simulink model "MotorDriveThermalTestbench"  (R2024b)
settings: Solver=daessc  StartTime=0.0  StopTime=2400  FixedStep=dt  RelTol=1e-3  AbsTol=1e-3
PreLoadFcn:
  | % Simulation parameters
  | MotorDriveThermalTestBenchParams;
model workspace (MAT data in the model file):
  V_frac_bridge = 0.0437
  V_fract_teeth = 0.9563
values from neighbouring files (symbols this model uses):
  CaseParams = struct()    [InverterThermalParams.m]
  HeatsinkParams = struct()    [InverterThermalParams.m]
undefined symbols (not defined in the file or in its folder): electricDrive, H_AH, H_AL, H_BH, H_BL, H_CH, H_CL, PipeParams, vehicleThermal
libraries: fl_lib x171, ee_lib x31, nesl_utility x28, nesl_utility_internal x12, sdl_lib x6, SimscapeFluids_lib x3, autolibshared x1
(part 1 of 4)
Description:
  | Copyright 2022 - 2023 The MathWorks, Inc.
settings Model: Creator=The MathWorks, Inc.  LastModifiedBy=jjha
settings SolverCC: AutoScaleAbsTol=off  InitialStep=1e-3  MaxConsecutiveMinStep=100  AlgebraicLoopSolver=TrustRegion
settings DataIOCC: MaxDataPoints=30000  SaveFormat=Array  SignalLoggingName=logsoutPMSMThermalTestbench  ReturnWorkspaceOutputsName=simoutPmsmThermalTestbench
settings OptimizationCC: BlockReduction=off  BooleanDataType=off  ReuseModelBlockBuffer=off  LifeSpan=inf
settings DebuggingCC: SaveWithParameterizedLinksMsg=none  SignalResolutionControl=TryResolveAllWithWarning  UnconnectedInputMsg=warning  UnconnectedOutputMsg=warning  UnconnectedLineMsg=warning  AllowSymbolicDim=off  SFUnexpectedBacktrackingDiag=warning  SFNoUnconditionalDefaultTransitionDiag=warning  SFExecutionAtInitializationDiag=none  ArithmeticOperatorsInVariantConditions=warning
settings HardwareCC: ProdBitPerPointer=32  ProdBitPerSizeT=32  ProdBitPerPtrDiffT=32  ProdLargestAtomicFloat=None  ProdIntDivRoundTo=Undefined  ProdEndianess=Unspecified  ProdWordSize=32  ProdHWDeviceType=32-bit Generic  TargetUnknown=on
settings ModelReferenceCC: EnableRefExpFcnMdlSchedulingChecks=on  PropagateSignalLabelsOutOfModel=off
settings SFSimCC: SimUseLocalCustomCode=off  CustomCodeUndefinedFunction=UseInterfaceOnly
settings RTWCC: RTWUseLocalCustomCode=off  GPUComputeCapability=3.5  DLArmComputeVersion=19.05
settings CodeAppCC: StateflowObjectComments=on
settings GRTTargetCC: TargetLangStandard=C89/C90 (ANSI)
settings ConfigComp: CovMetricSettings=dw  CovSaveCumulativeToWorkspaceVar=on  CovSaveSingleToWorkspaceVar=on  CovExternalEMLEnable=off  CovSFcnEnable=off
settings SimscapeCC: SimscapeLogType=all  SimscapeLogSimulationStatistics=on  SimscapeLogName=simlogPmsmThermalTestbench  SimscapeLogLimitData=off  SimscapeLogDataHistory=30000

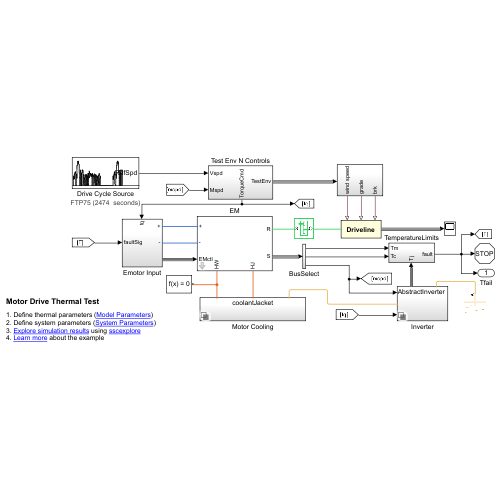
[thumbnail: Simulink's stored preview of the top-level diagram]
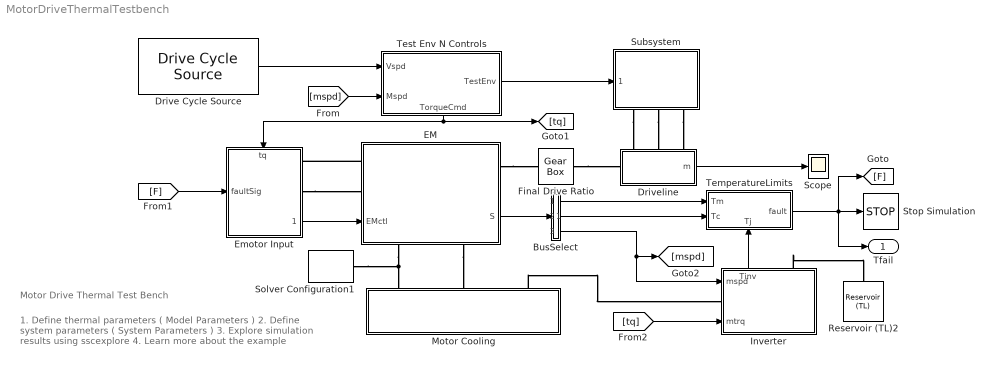
== system MotorDriveThermalTestbench ==
  note: Motor Drive Thermal Test Bench
  note: 1. Define thermal parameters ( Model Parameters )
      | 2. Define system parameters ( System Parameters )
      | 3. Explore simulation results using sscexplore
      | 4. Learn more about the example
  BusSelect : Subsystem
  Drive Cycle Source : autolibshared/Drive Cycle Source  cycleVar=FTP75  wsVar=LSHT  fileVar=cycleFTP75.mat  tfinal="2474  seconds"  cycleRepeat=off  outAccPort=off  outGearPort=off  gearList=No gear data  t_wot1=5  xdot_woto=0  xdot_wot1=30  t_wot2=20  xdot_wot2=0  t_wotend=30  srcUnit=m/s  outUnit=km/h  srcAccUnit=m/s/s  outAccUnit=m/s^2  dt=0  aMode=1  faultOption=off  velBnd=2  velBndUnit=mph  inUnit=m/s  timeBnd=1  failOption=off  stopSim=off  maxFaultCnt=10  maxFaultTime=2  maxTotFaultTime=15  traceOption=off  dtTrace=1  traceWindow=10  lastDCname=FTP75  lastOutUnit=mph  lastDT=0  lastTB=1  lastSB=2  forceCalcBound=off
  Driveline : Subsystem
      settings: PortSchema="{\"entries\":[{\"content\":{\"sides\":[{\"content\":{\"connectorIds\":[\"Out1\"]},\"type\":\"ConnectorPlacement.EquallySpacedRectSide\",\"uuid\":\"f321ff85-78a4-45a4-ab97-f20c5abfaf5e\"},{\"content\":{\"connectorIds\":[\"RConn1\"],\"side\":\"RIGHT\"},\"type\":\"ConnectorPlacement.EquallySpacedRectSide\",\"uuid\":\"2baf3540-3ef2-4140-8c68-0a1895e3ee25\"},{\"content\":{\"connectorIds\":[\"LConn1\",\"LConn2\",\"LConn3\"],\"side\":\"TOP\"},\"type\":\"ConnectorPlacement.EquallySpacedRectSide\",\"uuid\":\"1e5b09ba-71c5-41d6-b265-2fb2d783e941\"}]},\"type\":\"ConnectorPlacement.EquallySpacedConnector\",\"uuid\":\"4c01441a-ee4a-4858-900a-4caacc6910c3\"}],\"packageUris\":[\"http://schema.mathworks.com/mf0/Connector/R2020b\"],\"version\":\"1.0\"}"
      mask Display:
      | %disp(get_param(gcb, 'Name'))
      | disp(['{\bf\fontsize{12}' get_param(gcb, 'Name') '}'], 'texmode','on');
  EM : Subsystem  mask{InitTemp=vehicleThermal.coolant_T_init, IronSpHeat=electricDrive.IronSpHeat, CopperSpHeat=electricDrive.CopperSpHeat, IronThConductivity=electricDrive.IronThConductivity, GrossToothMass=electricDrive.MotorThermal.GrossToothMass, WindingMass=electricDrive.MotorThermal.WindingMass, max_torque=electricDrive.max_torque, max_power=electricDrive.max_power, Tctc=electricDrive.Tctc, spMat=electricDrive.motor_loss_map.spMat, tqMat=electricDrive.motor_loss_map.tqMat, lossMat=electricDrive.motor_loss_map.lossMat, StatorBackIronMass=electricDrive.MotorThermal.StatorBackIronMass, StatorRootDia=electricDrive.MotorThermal.StatorRootDia, stator_od=electricDrive.MotorThermal.stator_od, StatorWindingOhArea=electricDrive.MotorThermal.StatorWindingOhArea, Bridgemass=electricDrive.MotorThermal.Bridgemass, rotor_od=electricDrive.MotorThermal.rotor_od, rotorStackLength=electricDrive.MotorThermal.rotorStackLength, RotorBackIronMass=electricDrive.MotorThermal.RotorBackIronMass, RotorAreaER=electricDrive.MotorThermal.RotorAreaER, RotorAreaCyl=electricDrive.MotorThermal.RotorAreaCyl}
      mask prompts: InitTemp "Initial Temperature(K)"; IronSpHeat "Specific Heat Iron(J/(K*kg))"; CopperSpHeat "Specific Heat Copper(J/(K*kg))"; IronThConductivity "Thermal Conductivity Iron(W/(K*m))"; GrossToothMass "Stator Teeth Mass(kg)"; WindingMass "Stator Winding Mass(kg)"; max_torque "Max Torque"; max_power "Max Power"; Tctc "Torque Control Time Constant"; spMat "Speed Vector (rpm)"; tqMat "TorqueVector (Nm)"; lossMat "Losses (W)"; StatorBackIronMass "Stator Back Iron Mass(kg)"; StatorRootDia "Stator Inner Diameter (m)"; stator_od "Stator Outer Diameter(m)"; StatorWindingOhArea "Stator Winding Area(m^2)"; Bridgemass "Magnet Mass(kg)"; rotor_od "Rotor Outer Diameter(m)"; rotorStackLength "Stack Length(m)"; RotorBackIronMass "Rotor Iron Mass(kg)"; RotorAreaER "Rotor Area ER(m^2)"; RotorAreaCyl "Rotor Cylinder Area(m^2)"
      settings: LibrarySourceBlock=EmotorLib/Emotor Thermal  PortSchema="{\"entries\":[{\"content\":{\"sides\":[{\"content\":{\"connectorIds\":[\"LConn1\",\"LConn2\",\"In1\"]},\"type\":\"ConnectorPlacement.EquallySpacedRectSide\",\"uuid\":\"10df522d-563d-4b08-8533-b994fdc6485c\"},{\"content\":{\"connectorIds\":[\"RConn1\",\"Out1\"],\"side\":\"RIGHT\"},\"type\":\"ConnectorPlacement.EquallySpacedRectSide\",\"uuid\":\"49c7f672-865f-471b-9e0c-89a8670e12b9\"},{\"content\":{\"connectorIds\":[],\"side\":\"TOP\"},\"type\":\"ConnectorPlacement.EquallySpacedRectSide\",\"uuid\":\"483d1bb0-f2a2-4e3e-b03d-59043e33c561\"},{\"content\":{\"connectorIds\":[\"RConn2\",\"RConn3\"],\"side\":\"BOTTOM\"},\"type\":\"ConnectorPlacement.EquallySpacedRectSide\",\"uuid\":\"9824884f-8ef8-4acd-9b94-f9f251c18df1\"}]},\"type\":\"ConnectorPlacement.EquallySpacedConnector\",\"uuid\":\"fbb57d51-9a3c-403f-b1bb-2fd61ef310af\"}],\"packageUris\":[\"http://schema.mathworks.com/mf0/Connector/R2020b\"],\"version\":\"1.0\"}"
      mask DialogControl Container5 Prompt: Electrical Parameters
      mask DialogControl ElecTorque Prompt: Electrical Torque Parameters
      mask DialogControl ElecLosses Prompt: Electrical Losses Parameter
      mask DialogControl Container6 Prompt: Thermal Parameters
      mask DialogControl Container8 Prompt: Rotor
      mask DialogControl Container7 Prompt: Stator
  Emotor Input : Subsystem
      settings: PortSchema="{\"entries\":[{\"content\":{\"sides\":[{\"content\":{\"connectorIds\":[\"In1\"]},\"type\":\"ConnectorPlacement.EquallySpacedRectSide\",\"uuid\":\"c4c07ff1-e6b7-44ff-b3a5-b0e10b4cc465\"},{\"content\":{\"connectorIds\":[\"RConn1\",\"RConn2\",\"Out1\"],\"side\":\"RIGHT\"},\"type\":\"ConnectorPlacement.EquallySpacedRectSide\",\"uuid\":\"925c4aa1-6eb7-46da-8525-6fdd9359c532\"},{\"content\":{\"connectorIds\":[\"In2\"],\"side\":\"TOP\"},\"type\":\"ConnectorPlacement.EquallySpacedRectSide\",\"uuid\":\"640b893a-14a3-4b76-a9bc-18e7c0276558\"}]},\"type\":\"ConnectorPlacement.EquallySpacedConnector\",\"uuid\":\"1af614e2-1b17-4f3a-ad07-bd248b373d7b\"}],\"packageUris\":[\"http://schema.mathworks.com/mf0/Connector/R2020b\"],\"version\":\"1.0\"}"
  Final Drive Ratio : fl_lib/Mechanical/Mechanisms/Gear Box  ratio=electricDrive.VehicleParams.Gear_ratio  t_in_specify=off  t_in_priority=High  t_in=0 N*m  t_in_nominal_specify=off  t_in_nominal_value=1  t_in_nominal_unit=N*m  t_out_specify=off  t_out_priority=High  t_out=0 N*m  t_out_nominal_specify=off  t_out_nominal_value=1  t_out_nominal_unit=N*m
  Inverter : Subsystem  Variant=on  VariantControlMode=label  LabelModeActiveChoice=AbstractOn
      settings: PortSchema="{\"entries\":[{\"content\":{\"sides\":[{\"content\":{\"connectorIds\":[\"In1\",\"LConn1\",\"In2\"]},\"type\":\"ConnectorPlacement.EquallySpacedRectSide\",\"uuid\":\"633c2257-0ab1-4a3f-bc19-db971bbd7d23\"},{\"content\":{\"connectorIds\":[],\"side\":\"RIGHT\"},\"type\":\"ConnectorPlacement.EquallySpacedRectSide\",\"uuid\":\"268aca27-453a-4262-b99b-2b00bb036744\"},{\"content\":{\"connectorIds\":[\"Out1\",\"LConn2\"],\"side\":\"TOP\"},\"type\":\"ConnectorPlacement.EquallySpacedRectSide\",\"uuid\":\"94eb7410-69a0-4bb3-bfbc-11fdf2441086\"}]},\"type\":\"ConnectorPlacement.EquallySpacedConnector\",\"uuid\":\"4856a95d-ab29-4fb1-a283-1ba036af507a\"}],\"packageUris\":[\"http://schema.mathworks.com/mf0/Connector/R2020b\"],\"version\":\"1.0\"}"
  Motor Cooling : Subsystem  Variant=on  VariantControlMode=label  LabelModeActiveChoice=JacketOn
      settings: PortSchema="{\"entries\":[{\"content\":{\"sides\":[{\"content\":{\"connectorIds\":[]},\"type\":\"ConnectorPlacement.EquallySpacedRectSide\",\"uuid\":\"fad2e2e2-c8a8-4ae7-a5e0-e2d04801ad81\"},{\"content\":{\"connectorIds\":[],\"side\":\"RIGHT\"},\"type\":\"ConnectorPlacement.EquallySpacedRectSide\",\"uuid\":\"a876eae4-26d9-44a3-9dd3-410a35dafbf1\"},{\"content\":{\"connectorIds\":[\"LConn1\",\"LConn2\",\"LConn3\"],\"side\":\"TOP\"},\"type\":\"ConnectorPlacement.EquallySpacedRectSide\",\"uuid\":\"b2d352a8-e78b-4f23-87e4-b1c134d4f518\"}]},\"type\":\"ConnectorPlacement.EquallySpacedConnector\",\"uuid\":\"4da0a1ca-7739-4d5f-a9bc-f50bcf2d911d\"}],\"packageUris\":[\"http://schema.mathworks.com/mf0/Connector/R2020b\"],\"version\":\"1.0\"}"
  Reservoir (TL)2 : fl_lib/Thermal Liquid/Elements/Reservoir (TL)  pressure_spec=foundation.enum.pressure_spec.atmospheric  reservoir_pressure=0.101325 MPa  reservoir_temperature=TankParams.Temp K  area=0.01 m^2
  Scope : Scope
  Solver Configuration1 : nesl_utility/Solver Configuration  PhysicalDomain=network_engine_domain  SubClassName=solver  LeftPortType=input  RightPortType=generic  Tones=[]  Harmonics=[]  SimulateNoise=off  Profile=off  UseLocalSampling=off  EnableSwitchedLinearOptims=on  FrequencyDomain=off  UseCCode=off  RelTol=0.001  AbsTol=0.001  MinStep=1e-09  ToWorkspace=off  RevertToSquareIcSolve=off  NumHomotopyIterations=100  PhasorMode=off  PhasorModeNumHarmonics=1  ConsistencySolver=NEWTON_XTOL_AFTER_FTOL  IndexReductionMethod=DerivativeReplacement  DoDC=off  ResidualTolerance=1e-09  ConsistencyTolSource=GLOBAL  ConsistencyAbsTol=0.001  ConsistencyRelTol=0.001  ConsistencyTolFactor=0.001  UseLocalSolver=off  LocalSolverChoice=NE_BACKWARD_EULER_ADVANCER  ResolveIndetEquations=on  FunctionEvalNumThread=1  LocalSolverSampleTime=0.001  DoFixedCost=off  MaxNonlinIter=3  MaxModeIter=2  ComputeImpulses=off  ImpulseIterations=2  LinearAlgebra=auto  LinearAlgebraNumThread=0  EquationFormulation=NE_TIME_EF  DelaysMemoryBudget=1024  AutomaticFiltering=on  FilteringTimeConstant=0.001  PartitionStorageMethod=AS_NEEDED  PartitionMemoryBudget=1024  PartitionMethod=ROBUST  MultibodyUseLocalSolver=off  MultibodyLocalSolverChoice=ODE1  MultibodyLocalSolverSampleTime=0.001
  Stop Simulation : Stop
  Subsystem : Subsystem
      settings: PortSchema="{\"entries\":[{\"content\":{\"sides\":[{\"content\":{\"connectorIds\":[]},\"type\":\"ConnectorPlacement.EquallySpacedRectSide\",\"uuid\":\"5b33bb33-1028-4467-9d0b-860d7c65cb16\"},{\"content\":{\"connectorIds\":[\"RConn1\",\"RConn2\",\"RConn3\"],\"side\":\"RIGHT\"},\"type\":\"ConnectorPlacement.EquallySpacedRectSide\",\"uuid\":\"d30bcb89-569c-4584-a5e8-bf96143649ac\"},{\"content\":{\"connectorIds\":[\"In1\"],\"side\":\"TOP\"},\"type\":\"ConnectorPlacement.EquallySpacedRectSide\",\"uuid\":\"a556bd16-04f6-4e3c-9a78-edea790b19fa\"}]},\"type\":\"ConnectorPlacement.EquallySpacedConnector\",\"uuid\":\"7b9502e3-af00-49d8-8813-697019fc00d4\"}],\"packageUris\":[\"http://schema.mathworks.com/mf0/Connector/R2020b\"],\"version\":\"1.0\"}"
  TemperatureLimits : Subsystem
      settings: PortSchema="{\"entries\":[{\"content\":{\"sides\":[{\"content\":{\"connectorIds\":[\"In1\",\"In2\"]},\"type\":\"ConnectorPlacement.EquallySpacedRectSide\",\"uuid\":\"44686035-e0c2-483b-a3a4-d0f17b02753c\"},{\"content\":{\"connectorIds\":[\"Out1\"],\"side\":\"RIGHT\"},\"type\":\"ConnectorPlacement.EquallySpacedRectSide\",\"uuid\":\"194b74d6-8594-4ad9-8d93-17205dccb996\"},{\"content\":{\"connectorIds\":[],\"side\":\"TOP\"},\"type\":\"ConnectorPlacement.EquallySpacedRectSide\",\"uuid\":\"c06a3734-ddd3-437f-914d-d266a0b88b6a\"},{\"content\":{\"connectorIds\":[\"In3\"],\"side\":\"BOTTOM\"},\"type\":\"ConnectorPlacement.EquallySpacedRectSide\",\"uuid\":\"63fcb3ec-4e8f-48a9-87ba-5ecb026b4494\"}]},\"type\":\"ConnectorPlacement.EquallySpacedConnector\",\"uuid\":\"f21c992b-3b0c-41f1-8f0e-ab867b6bfe49\"}],\"packageUris\":[\"http://schema.mathworks.com/mf0/Connector/R2020b\"],\"version\":\"1.0\"}"
  Test Env N Controls : Subsystem
      settings: PortSchema="{\"entries\":[{\"content\":{\"sides\":[{\"content\":{\"connectorIds\":[\"In1\",\"In2\"]},\"type\":\"ConnectorPlacement.EquallySpacedRectSide\",\"uuid\":\"bc333059-d3e6-4874-bec1-9f2659eeb99d\"},{\"content\":{\"connectorIds\":[\"Out1\"],\"side\":\"RIGHT\"},\"type\":\"ConnectorPlacement.EquallySpacedRectSide\",\"uuid\":\"65f46e5f-0102-4820-9504-ef274ed3cc10\"},{\"content\":{\"connectorIds\":[],\"side\":\"TOP\"},\"type\":\"ConnectorPlacement.EquallySpacedRectSide\",\"uuid\":\"27b5bec7-80ae-4482-837c-96dbc3d5f31c\"},{\"content\":{\"connectorIds\":[\"Out2\"],\"side\":\"BOTTOM\"},\"type\":\"ConnectorPlacement.EquallySpacedRectSide\",\"uuid\":\"d5fa4694-16ae-4ec4-a358-749ebe1665d7\"}]},\"type\":\"ConnectorPlacement.EquallySpacedConnector\",\"uuid\":\"e3722406-f8ed-4051-ae00-9576266ee651\"}],\"packageUris\":[\"http://schema.mathworks.com/mf0/Connector/R2020b\"],\"version\":\"1.0\"}"
  Tfail : Outport
  wires:
  Driveline/1(m) -> Scope/1
  Test Env N Controls/1(TestEnv) -> Subsystem/1(" ")
  Drive Cycle Source/1 -> Test Env N Controls/1(Vspd)
  Test Env N Controls/2(TorqueCmd) -> Emotor Input/2(tq), [tq]
  [mspd] -> Test Env N Controls/2(Mspd)
  [F] -> Emotor Input/1(faultSig)
  [tq] -> Inverter/2(mtrq)
  Inverter/1(Tinv) -> TemperatureLimits/3(Tj)
  TemperatureLimits/1(fault) -> Tfail/1, [F], Stop Simulation/1
  BusSelect/3(<EM1rpm>) -> Inverter/1(mspd), [mspd]
  EM/1(S) -> BusSelect/1(In1)
  BusSelect/1(<Tmag>) -> TemperatureLimits/1(Tm)
  BusSelect/2(<Tcoil>) -> TemperatureLimits/2(Tc)
  Emotor Input/1(" ") -> EM/1(EMctl)
  connections:
  Final Drive Ratio/RConn1 -- Driveline/RConn1
  EM/RConn1 -- Final Drive Ratio/LConn1
  EM/RConn3 -- Motor Cooling/LConn2
  Inverter/LConn2 -- Reservoir (TL)2/LConn1
  Subsystem/RConn2 -- Driveline/LConn2
  Subsystem/RConn1 -- Driveline/LConn3
  Subsystem/RConn3 -- Driveline/LConn1
  Solver Configuration1/RConn1 -- EM/RConn2 -- Motor Cooling/LConn1
  Motor Cooling/LConn3 -- Inverter/LConn1
  EM/LConn1 -- Emotor Input/RConn1
  Emotor Input/RConn2 -- EM/LConn2

== system MotorDriveThermalTestbench/BusSelect ==
  In1 : Inport
  Bus Selector : BusSelector  OutputSignals=magT,coilT,EMrpm
  <Tmag> : Outport
  <Tcoil> : Outport  Port=2
  <EM1rpm> : Outport  Port=3
  wires:
  In1/1 -> Bus Selector/1
  Bus Selector/2 -> <Tcoil>/1  "<coilT>"
  Bus Selector/3 -> <EM1rpm>/1  "<EMrpm>"
  Bus Selector/1 -> <Tmag>/1  "<magT>"

== system MotorDriveThermalTestbench/Driveline ==
  Brake Rear : sdl_lib/Brakes & Detents/Rotational/Disc Brake  r_mean=150 mm  bore=10 mm  n_pads=2  thermal_port=simscape.enum.thermaleffects.omit  mu_static=0.9  mu_coulomb=0.7  temperature_TLU=[280, 300, 320] K  mu_static_TLU=[.9, .8, .7]  mu_coulomb_TLU=[.8, .7, .6]  brkwy_vel=0.1 rad/s  visc_coef=0 N*m*s/rad  thermal_mass=50 kJ/K  temperature_specify=off  temperature_priority=High  temperature=300 K  temperature_nominal_specify=off  temperature_nominal_value=1  temperature_nominal_unit=K
  PS-Simulink Converter1 : nesl_utility/PS-Simulink Converter  PhysicalDomain=network_engine_domain  SubClassName=ps_output  LeftPortType=input  RightPortType=output  PseudoPeriodic=off  Frequencies=[]  VectorFormat=inherit  Unit=inherit  AffineConversion=off
  Tire FL : sdl_lib/Tires & Vehicles/Tire (Magic Formula)  parameterization=sdl.enum.magic_tire_model.peak  F_z1=3000 N  F_x1=3500 N  kappa1=10  B_m=10  C_m=1.9  D_m=1  E_m=0.97  fz0=4000 N  p_Cx=1.685  p_Dx=[1.21, -.037]  p_Ex=[.344, .095, -.02, 0]  p_Kx=[21.51, -.163, .245]  p_Hx=[-.002, .002]  p_Vx=[0, 0]  rolling_radius_model=sdl.enum.RollingRadiusParameterization.Constant  r_e="driveline.tireRollingRadius_cm  cm"  r_0=0.3 m  breff=8.39  dreff=0.26  freff=0.074  q_re0=0.99  q_v1=0.008  longvl=17 m/s  cz=5e5 N/m  model_resistance=simscape.enum.onoff.off  resistance_model=sdl.enum.rollingResistanceParameterization.constant  coeff=0.015  p_tire=250e3 Pa  alpha=-0.003  beta=0.97  coeff_a=84e-4  coeff_b=6.2e-4 s/m  coeff_c=1.6e-4 s^2/m^2  p_tire0=240e3 Pa  fz0_resistance=4000 N  vH0=16 m/s  q_Sy=[.0082, 0, .0014, .001, 0, 0, 1.08, -.5]  v_thr=0.001 m/s  enable_scaling_coefficients=false  lfzO=1  lcx=1  lmux=1  lex=1  lkx=1  lhx=1  lvx=1  lmy=1  model_compliance=sdl.enum.compliance.off  stiffness=1e6 N/m  damping=1000 N*s/m  model_inertia=sdl.enum.model_inertia.off  inertia=1 kg*m^2  initial_velocity=0 rad/s  vxlow=0.1 m/s  v_tr_thr=0.1*(0.1) m/s  kpumin=-1e5  kpumax=1e5
  Tire FR : sdl_lib/Tires & Vehicles/Tire (Magic Formula)  parameterization=sdl.enum.magic_tire_model.peak  F_z1=3000 N  F_x1=3500 N  kappa1=10  B_m=10  C_m=1.9  D_m=1  E_m=0.97  fz0=4000 N  p_Cx=1.685  p_Dx=[1.21, -.037]  p_Ex=[.344, .095, -.02, 0]  p_Kx=[21.51, -.163, .245]  p_Hx=[-.002, .002]  p_Vx=[0, 0]  rolling_radius_model=sdl.enum.RollingRadiusParameterization.Constant  r_e="driveline.tireRollingRadius_cm  cm"  r_0=0.3 m  breff=8.39  dreff=0.26  freff=0.074  q_re0=0.99  q_v1=0.008  longvl=17 m/s  cz=5e5 N/m  model_resistance=simscape.enum.onoff.off  resistance_model=sdl.enum.rollingResistanceParameterization.constant  coeff=0.015  p_tire=250e3 Pa  alpha=-0.003  beta=0.97  coeff_a=84e-4  coeff_b=6.2e-4 s/m  coeff_c=1.6e-4 s^2/m^2  p_tire0=240e3 Pa  fz0_resistance=4000 N  vH0=16 m/s  q_Sy=[.0082, 0, .0014, .001, 0, 0, 1.08, -.5]  v_thr=0.001 m/s  enable_scaling_coefficients=false  lfzO=1  lcx=1  lmux=1  lex=1  lkx=1  lhx=1  lvx=1  lmy=1  model_compliance=sdl.enum.compliance.off  stiffness=1e6 N/m  damping=1000 N*s/m  model_inertia=sdl.enum.model_inertia.off  inertia=1 kg*m^2  initial_velocity=0 rad/s  vxlow=0.1 m/s  v_tr_thr=0.1*(0.1) m/s  kpumin=-1e5  kpumax=1e5
  Tire RL : sdl_lib/Tires & Vehicles/Tire (Magic Formula)  parameterization=sdl.enum.magic_tire_model.peak  F_z1=3000 N  F_x1=3500 N  kappa1=10  B_m=10  C_m=1.9  D_m=1  E_m=0.97  fz0=4000 N  p_Cx=1.685  p_Dx=[1.21, -.037]  p_Ex=[.344, .095, -.02, 0]  p_Kx=[21.51, -.163, .245]  p_Hx=[-.002, .002]  p_Vx=[0, 0]  rolling_radius_model=sdl.enum.RollingRadiusParameterization.Constant  r_e="driveline.tireRollingRadius_cm  cm"  r_0=0.3 m  breff=8.39  dreff=0.26  freff=0.074  q_re0=0.99  q_v1=0.008  longvl=17 m/s  cz=5e5 N/m  model_resistance=simscape.enum.onoff.off  resistance_model=sdl.enum.rollingResistanceParameterization.constant  coeff=0.015  p_tire=250e3 Pa  alpha=-0.003  beta=0.97  coeff_a=84e-4  coeff_b=6.2e-4 s/m  coeff_c=1.6e-4 s^2/m^2  p_tire0=240e3 Pa  fz0_resistance=4000 N  vH0=16 m/s  q_Sy=[.0082, 0, .0014, .001, 0, 0, 1.08, -.5]  v_thr=0.001 m/s  enable_scaling_coefficients=false  lfzO=1  lcx=1  lmux=1  lex=1  lkx=1  lhx=1  lvx=1  lmy=1  model_compliance=sdl.enum.compliance.off  stiffness=1e6 N/m  damping=1000 N*s/m  model_inertia=sdl.enum.model_inertia.off  inertia=1 kg*m^2  initial_velocity=0 rad/s  vxlow=0.1 m/s  v_tr_thr=0.1*(0.1) m/s  kpumin=-1e5  kpumax=1e5
  Tire RR : sdl_lib/Tires & Vehicles/Tire (Magic Formula)  parameterization=sdl.enum.magic_tire_model.peak  F_z1=3000 N  F_x1=3500 N  kappa1=10  B_m=10  C_m=1.9  D_m=1  E_m=0.97  fz0=4000 N  p_Cx=1.685  p_Dx=[1.21, -.037]  p_Ex=[.344, .095, -.02, 0]  p_Kx=[21.51, -.163, .245]  p_Hx=[-.002, .002]  p_Vx=[0, 0]  rolling_radius_model=sdl.enum.RollingRadiusParameterization.Constant  r_e="driveline.tireRollingRadius_cm  cm"  r_0=0.3 m  breff=8.39  dreff=0.26  freff=0.074  q_re0=0.99  q_v1=0.008  longvl=17 m/s  cz=5e5 N/m  model_resistance=simscape.enum.onoff.off  resistance_model=sdl.enum.rollingResistanceParameterization.constant  coeff=0.015  p_tire=250e3 Pa  alpha=-0.003  beta=0.97  coeff_a=84e-4  coeff_b=6.2e-4 s/m  coeff_c=1.6e-4 s^2/m^2  p_tire0=240e3 Pa  fz0_resistance=4000 N  vH0=16 m/s  q_Sy=[.0082, 0, .0014, .001, 0, 0, 1.08, -.5]  v_thr=0.001 m/s  enable_scaling_coefficients=false  lfzO=1  lcx=1  lmux=1  lex=1  lkx=1  lhx=1  lvx=1  lmy=1  model_compliance=sdl.enum.compliance.off  stiffness=1e6 N/m  damping=1000 N*s/m  model_inertia=sdl.enum.model_inertia.off  inertia=1 kg*m^2  initial_velocity=0 rad/s  vxlow=0.1 m/s  v_tr_thr=0.1*(0.1) m/s  kpumin=-1e5  kpumax=1e5
  Vehicle Body : sdl_lib/Tires & Vehicles/Vehicle Body  mass=driveline.vehMass_kg kg  n_w=2  x_f=1.4 m  x_r=1.6 m  y_c=0.5 m  mass_var=simscape.enum.onoff.off  g=9.81 m/s^2  liftoff_warning=simscape.enum.onoff.off  area=3 m^2  Cd_var=false  Cd=0.4  rho=1.18 kg/m^3  model_pitch=simscape.enum.onoff.off  inertia=4000 kg*m^2  suspension_model=sdl.enum.linearTLU.linear  k_f=1e4 N/m  b_f=1e4 N*s/m  k_r=1e4 N/m  b_r=1e4 N*s/m  k_f_TLU=[-2000, -1000, 0, 1000, 2000] N  x_f_TLU=[-.4, -.2, 0, .2, .4] m  b_f_TLU=[-200, -100, 0, 100, 200] N  v_f_TLU=[-4, -2, 0, 2, 4] m/s  k_r_TLU=[-2000, -1000, 0, 1000, 2000] N  x_r_TLU=[-.4, -.2, 0, .2, .4] m  b_r_TLU=[-200, -100, 0, 100, 200] N  v_r_TLU=[-4, -2, 0, 2, 4] m/s  interp_method=simscape.enum.interpolation.linear  extrap_method=simscape.enum.extrapolation.linear  model_hardstop=simscape.enum.onoff.off  upper_bound_f=.25 m  lower_bound_f=-.25 m  stop_k_f=1e6 N/m  stop_b_f=150 N*s/m  upper_bound_r=.25 m  lower_bound_r=-.25 m  stop_k_r=1e6 N/m  stop_b_r=150 N*s/m  initial_pitch=0 rad  initial_pitch_rate=0 rad/s  v_specify=on  v_priority=High  v=0 kph  v_nominal_specify=on  v_nominal_value=1  v_nominal_unit=m/s
      settings: InternalSimscapePortConfiguration="{\"Bottom\":[{\"id\":\"NR\",\"label\":\"NR\",\"type\":\"output\"},{\"id\":\"NF\",\"label\":\"NF\",\"type\":\"output\"},{\"id\":\"beta\",\"label\":\"beta\",\"type\":\"input\"}],\"Left\":[{\"id\":\"H\",\"label\":\"H\",\"type\":\"foundation.mechanical.translational.translational\"}],\"Right\":[],\"Top\":[{\"id\":\"V\",\"label\":\"V\",\"type\":\"output\"},{\"id\":\"wind\",\"label\":\"W\",\"type\":\"input\"}]}"
  m/s to Km/hr : Gain  Gain=3.6
  brk : PMIOPort  Side=Left
  rodeGrd : PMIOPort  Port=2  Side=Left
  windSpd : PMIOPort  Port=3  Side=Left
  FA : PMIOPort  Port=4  Side=Right
  Bus Element Out : Outport  PortName=m  Element=VehSpd
  wires:
  m/s to Km/hr/1 -> Bus Element Out/1  "VehSpd"
  PS-Simulink Converter1/1 -> m/s to Km/hr/1
  connections:
  Brake Rear/LConn1 -- brk/RConn1
  Tire FR/RConn2 -- Tire RL/RConn2 -- Tire RR/RConn2 -- Vehicle Body/LConn1 -- Tire FL/RConn2
  Tire RL/LConn2 -- Tire RR/LConn2 -- Brake Rear/LConn2
  Tire FL/LConn2 -- FA/RConn1 -- Tire FR/LConn2
  PS-Simulink Converter1/LConn1 -- Vehicle Body/LConn2
  Tire RL/LConn1 -- Vehicle Body/RConn1 -- Tire RR/LConn1
  Vehicle Body/RConn2 -- Tire FR/LConn1 -- Tire FL/LConn1
  windSpd/RConn1 -- Vehicle Body/LConn3
  Vehicle Body/RConn3 -- rodeGrd/RConn1

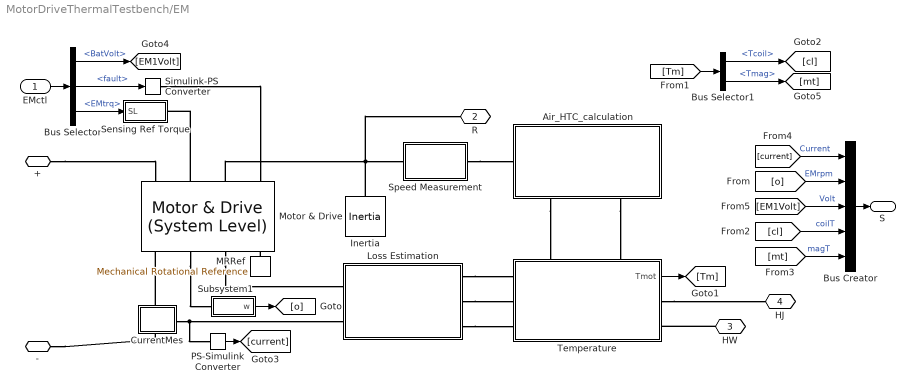
== system MotorDriveThermalTestbench/EM ==
  EMctl : Inport
  Air_HTC_calculation : Subsystem
      settings: PortSchema="{\"entries\":[{\"content\":{\"sides\":[{\"content\":{\"connectorIds\":[\"LConn1\"]},\"type\":\"ConnectorPlacement.EquallySpacedRectSide\",\"uuid\":\"c3fc49c2-0151-484f-b0d8-f4e4a060bcaf\"},{\"content\":{\"connectorIds\":[],\"side\":\"RIGHT\"},\"type\":\"ConnectorPlacement.EquallySpacedRectSide\",\"uuid\":\"c73251fe-fcad-4c5f-9d27-fb7ac98c9b31\"},{\"content\":{\"connectorIds\":[],\"side\":\"TOP\"},\"type\":\"ConnectorPlacement.EquallySpacedRectSide\",\"uuid\":\"06ea8515-c1b4-4445-9ea2-9a6fe3b8d822\"},{\"content\":{\"connectorIds\":[\"RConn1\",\"RConn2\"],\"side\":\"BOTTOM\"},\"type\":\"ConnectorPlacement.EquallySpacedRectSide\",\"uuid\":\"0d77474d-64a7-49ab-b2b5-eb3962b26dfa\"}]},\"type\":\"ConnectorPlacement.EquallySpacedConnector\",\"uuid\":\"651eda7a-2416-4496-9b8b-1b2d725cf6dd\"}],\"packageUris\":[\"http://schema.mathworks.com/mf0/Connector/R2020b\"],\"version\":\"1.0\"}"
  Bus Creator : BusCreator  Inputs=5
  Bus Selector : BusSelector  OutputSignals=BatVolt,fault,EMtrq
  Bus Selector1 : BusSelector  OutputSignals=Tcoil,Tmag
  CurrentMes : Subsystem
      settings: PortSchema="{\"entries\":[{\"content\":{\"sides\":[{\"content\":{\"connectorIds\":[\"LConn1\"]},\"type\":\"ConnectorPlacement.EquallySpacedRectSide\",\"uuid\":\"aec73178-3b68-40df-935a-7f5359bce9cd\"},{\"content\":{\"connectorIds\":[],\"side\":\"RIGHT\"},\"type\":\"ConnectorPlacement.EquallySpacedRectSide\",\"uuid\":\"aa898e43-8a60-4280-99e9-69a0b0908b52\"},{\"content\":{\"connectorIds\":[\"LConn2\"],\"side\":\"TOP\"},\"type\":\"ConnectorPlacement.EquallySpacedRectSide\",\"uuid\":\"450895ec-a170-4755-8b37-3fd418fe4f7c\"},{\"content\":{\"connectorIds\":[\"RConn1\"],\"side\":\"BOTTOM\"},\"type\":\"ConnectorPlacement.EquallySpacedRectSide\",\"uuid\":\"50e67d36-6ee8-4450-bc7a-5decbfd7b4fc\"}]},\"type\":\"ConnectorPlacement.EquallySpacedConnector\",\"uuid\":\"d52bc816-e8fd-442f-9361-ac497bbc1898\"}],\"packageUris\":[\"http://schema.mathworks.com/mf0/Connector/R2020b\"],\"version\":\"1.0\"}"
  Inertia : fl_lib/Mechanical/Rotational Elements/Inertia  inertia=0.02 kg*m^2  num_ports=foundation.enum.numPorts2.one  w_specify=on  w_priority=High  w=0 rad/s  w_nominal_specify=off  w_nominal_value=1  w_nominal_unit=rad/s  t_specify=off  t_priority=None  t=0 N*m  t_nominal_specify=off  t_nominal_value=1  t_nominal_unit=N*m
  Loss Estimation : Subsystem
  MRRef : fl_lib/Mechanical/Rotational Elements/Mechanical Rotational Reference
  Motor & Drive : ee_lib/Electromechanical/Motor & Drive (System Level)  torque_speed_param=2  overtorque_param=ee.enum.electromech.overtorque.no  T_t=[max_torque max_torque max_torque 0] N*m  T_t_intermittent=[.36, .32, .28, 0] N*m  T_t_2D=[.09, .09, .09; .08, .08, .08; .07, .07, .07; 0, 0, 0] N*m  T_t_intermittent_2D=[.36, .36, .36; .32, .32, .32; .28, .28, .28; 0, 0, 0] N*m  w_t=[ 0 3.75e+3 7.5e+3 8e+3 ] rpm  vdc_t=[6, 12, 24] V  torque_max=electricDrive.max_torque N*m  power_max=electricDrive.max_power W  torque_max_intermittent=0.4 N*m  power_max_intermittent=120 W  time_overtorque=30 s  time_recover=60 s  Tc=electricDrive.Tctc s  EnableSwitch=simscape.enum.onoff.on  losses_param=2  eff=96  w_eff=1500 rpm  T_eff=50 N*m  Piron=200 W  Pbase=0 W  w_eff_vec=electricDrive.motor_loss_map.spMat rpm  T_eff_vec="electricDrive.motor_loss_map.tqMat      N*m"  v_eff_vec=[100, 250, 400] V  losses_mat=electricDrive.motor_loss_map.lossMat W  efficiency_mat=[95 95 95 95; 95 95 95 95; 95 95 95 95; 95 95 95 95; 95 95 95 95]  losses_mat_3D=ones(5, 4, 3) W  efficiency_mat_3D=95 * ones(5, 4, 3)  Res=0 Ohm  J=0 kg*m^2  lam=1e-5 N*m/(rad/s)  speed0=0 rpm  fault_condition=1  fault_threshold=0.5  faulted_specify=off  faulted_priority=None  faulted=0  faulted_nominal_specify=off  faulted_nominal_value=1  faulted_nominal_unit=1  isSwitchedOff_specify=off  isSwitchedOff_priority=None  isSwitchedOff=0  isSwitchedOff_nominal_specify=off  isSwitchedOff_nominal_value=1  isSwitchedOff_nominal_unit=1  torqueLimitContinuous_specify=off  torqueLimitContinuous_priority=None  torqueLimitContinuous=0 N*m  torqueLimitContinuous_nominal_specify=off  torqueLimitContinuous_nominal_value=1  torqueLimitContinuous_nominal_unit=N*m  alpha=0.00393 1/K  Tmeas=298.15 degC  Tmeas2=398.15 degC  losses_mat_T2=electricDrive.motor_loss_map.lossMat W  efficiency_mat_T2=[95 95 95 95; 95 95 95 95; 95 95 95 95; 95 95 95 95; 95 95 95 95]  losses_mat_3D_T2=ones(5, 4, 3) W  efficiency_mat_3D_T2=95 * ones(5, 4, 3)  thermal_mass=15000 J/K  initial_temperature=298.15 K
      settings: InternalSimscapePortConfiguration="{\"Bottom\":[],\"Left\":[{\"id\":\"Vp\",\"label\":\"+\",\"type\":\"foundation.electrical.electrical\"},{\"id\":\"Tr\",\"label\":\"Tr\",\"type\":\"input\"},{\"id\":\"R\",\"label\":\"R\",\"type\":\"foundation.mechanical.rotational.rotational\"},{\"id\":\"F\",\"label\":\"SW\",\"type\":\"input\"}],\"Right\":[{\"id\":\"Vm\",\"label\":\"-\",\"type\":\"foundation.electrical.electrical\"},{\"id\":\"Omega\",\"label\":\"w\",\"type\":\"output\"},{\"id\":\"H\",\"label\":\"H\",\"type\":\"foundation.thermal.thermal\"},{\"id\":\"C\",\"label\":\"C\",\"type\":\"foundation.mechanical.rotational.rotational\"}],\"Top\":[]}"
  PS-Simulink Converter : nesl_utility/PS-Simulink Converter  PhysicalDomain=network_engine_domain  SubClassName=ps_output  LeftPortType=input  RightPortType=output  PseudoPeriodic=off  Frequencies=[]  VectorFormat=inherit  Unit=inherit  AffineConversion=off
  Sensing Ref Torque : Subsystem
      mask Display: disp('trqRef')
  Simulink-PS Converter : nesl_utility/Simulink-PS Converter  PhysicalDomain=network_engine_domain  SubClassName=ps_input  LeftPortType=input  RightPortType=output  PseudoPeriodic=off  Frequencies=[]  NoiseDistribution=none  NoiseParameters=[]  Unit=1  AffineConversion=off  FilteringAndDerivatives=provide  SimscapeFilterOrder=1  InputFilterTimeConstant=0.001  UdotUserProvided=0
  Speed Measurement : Subsystem
  Subsystem1 : Subsystem
      settings: PortSchema="{\"entries\":[{\"content\":{\"sides\":[{\"content\":{},\"type\":\"ConnectorPlacement.EquallySpacedRectSide\",\"uuid\":\"73dca2aa-f399-4eeb-9d48-20c826d2ded4\"},{\"content\":{\"side\":\"RIGHT\"},\"type\":\"ConnectorPlacement.EquallySpacedRectSide\",\"uuid\":\"ff117f44-2f45-4c10-9502-0d11ada2d007\"},{\"content\":{\"connectorIds\":[\"LConn1\"],\"side\":\"TOP\"},\"type\":\"ConnectorPlacement.EquallySpacedRectSide\",\"uuid\":\"808df778-70a2-4117-a4b0-06aebafa20a3\"},{\"content\":{\"connectorIds\":[\"Out1\"],\"side\":\"BOTTOM\"},\"type\":\"ConnectorPlacement.EquallySpacedRectSide\",\"uuid\":\"ea26dad2-5611-48d3-b3ad-420e5e152393\"}]},\"type\":\"ConnectorPlacement.EquallySpacedConnector\",\"uuid\":\"b8b92b14-f871-4df7-89f6-65702e38d2f7\"}],\"packageUris\":[\"http://schema.mathworks.com/mf0/Connector/R2020b\"],\"version\":\"1.0\"}"
  Temperature : Subsystem
      settings: PortSchema="{\"entries\":[{\"content\":{\"sides\":[{\"content\":{\"connectorIds\":[\"LConn1\",\"LConn2\",\"LConn3\"]},\"type\":\"ConnectorPlacement.EquallySpacedRectSide\",\"uuid\":\"fee72484-960d-4cd4-9296-e38678962aa1\"},{\"content\":{\"connectorIds\":[\"Out1\",\"RConn1\",\"RConn2\"],\"side\":\"RIGHT\"},\"type\":\"ConnectorPlacement.EquallySpacedRectSide\",\"uuid\":\"5fc115b4-63fd-47d3-871d-1c82ac52ac43\"},{\"content\":{\"connectorIds\":[\"LConn4\",\"LConn5\"],\"side\":\"TOP\"},\"type\":\"ConnectorPlacement.EquallySpacedRectSide\",\"uuid\":\"406f719a-f995-4122-9f35-24e8332a2e84\"},{\"content\":{\"connectorIds\":[],\"side\":\"BOTTOM\"},\"type\":\"ConnectorPlacement.EquallySpacedRectSide\",\"uuid\":\"14dc85e6-8157-4b38-8651-862ce77721cd\"}]},\"type\":\"ConnectorPlacement.EquallySpacedConnector\",\"uuid\":\"1dcc2b5d-90fd-40de-873d-99118eb86bdd\"}],\"packageUris\":[\"http://schema.mathworks.com/mf0/Connector/R2020b\"],\"version\":\"1.0\"}"
  + : PMIOPort  Side=Left
  R : PMIOPort  Port=2  Side=Right
  HW : PMIOPort  Port=3  Side=Right
  HJ : PMIOPort  Port=4  Side=Right
  - : PMIOPort  Port=5  Side=Left
  S : Outport
  wires:
  [o] -> Bus Creator/2  "EMrpm"
  Bus Selector1/2 -> [mt]  "<Tmag>"
  Bus Selector1/1 -> [cl]  "<Tcoil>"
  EMctl/1 -> Bus Selector/1
  [cl] -> Bus Creator/4  "coilT"
  [mt] -> Bus Creator/5  "magT"
  [current] -> Bus Creator/1  "Current"
  Bus Selector/1 -> [EM1Volt]  "<BatVolt>"
  Bus Creator/1 -> S/1
  Temperature/1(Tmot) -> [Tm]
  PS-Simulink Converter/1 -> [current]
  Bus Selector/2 -> Simulink-PS Converter/1  "<fault>"
  Subsystem1/1(w) -> [o]
  [Tm] -> Bus Selector1/1
  Bus Selector/3 -> Sensing Ref Torque/1(SL)  "<EMtrq>"
  [EM1Volt] -> Bus Creator/3  "Volt"
  connections:
  Motor & Drive/RConn3 -- Loss Estimation/LConn1
  Simulink-PS Converter/RConn1 -- Motor & Drive/LConn4
  HW/RConn1 -- Temperature/RConn2
  -/RConn1 -- CurrentMes/RConn1
  Air_HTC_calculation/RConn1 -- Temperature/LConn4
  Motor & Drive/LConn2 -- Sensing Ref Torque/RConn1
  Motor & Drive/RConn2 -- Subsystem1/LConn1
  Speed Measurement/RConn1 -- Air_HTC_calculation/LConn1
  Loss Estimation/RConn1 -- Temperature/LConn1
  Loss Estimation/RConn2 -- Temperature/LConn2
  MRRef/LConn1 -- Motor & Drive/RConn4
  CurrentMes/LConn2 -- Motor & Drive/RConn1
  Temperature/RConn1 -- HJ/RConn1
  +/RConn1 -- Motor & Drive/LConn1
  Loss Estimation/RConn3 -- Temperature/LConn3
  Air_HTC_calculation/RConn2 -- Temperature/LConn5
  CurrentMes/LConn1 -- PS-Simulink Converter/LConn1 -- Loss Estimation/LConn2
  Motor & Drive/LConn3 -- Speed Measurement/LConn1 -- Inertia/LConn1 -- R/RConn1

== system MotorDriveThermalTestbench/Emotor Input ==
  faultSig : Inport
  tq : Inport  Port=2
  Bus Creator : BusCreator  Inputs=3
  Controlled Voltage Source : fl_lib/Electrical/Electrical Sources/Controlled Voltage Source
  Demux : Demux  Outputs=2
  Electrical Reference : fl_lib/Electrical/Electrical Elements/Electrical Reference
  PS Constant : fl_lib/Physical Signals/Sources/PS Constant  constant=electricDrive.Vnom V
  PS-Simulink Converter : nesl_utility/PS-Simulink Converter  PhysicalDomain=network_engine_domain  SubClassName=ps_output  LeftPortType=input  RightPortType=output  PseudoPeriodic=off  Frequencies=[]  VectorFormat=inherit  Unit=inherit  AffineConversion=off
  Terminator : Terminator
  + : PMIOPort  Side=Right
  - : PMIOPort  Port=2  Side=Right
  " " : Outport
  wires:
  tq/1 -> Bus Creator/2  "EMtrq"
  PS-Simulink Converter/1 -> Bus Creator/3  "BatVolt"
  Bus Creator/1 -> " "/1
  faultSig/1 -> Demux/1  "fault"
  Demux/1 -> Bus Creator/1  "fault"
  Demux/2 -> Terminator/1
  connections:
  PS Constant/RConn1 -- Controlled Voltage Source/RConn1 -- PS-Simulink Converter/LConn1
  Controlled Voltage Source/LConn1 -- +/RConn1
  -/RConn1 -- Electrical Reference/LConn1 -- Controlled Voltage Source/RConn2

== system MotorDriveThermalTestbench/Inverter ==
  mspd : Inport
  mtrq : Inport  Port=2
  "AbstractInverter " : Subsystem  VariantControl=AbstractOn
      settings: PortSchema="{\"entries\":[{\"content\":{\"sides\":[{\"content\":{\"connectorIds\":[\"In1\",\"In2\",\"LConn1\"]},\"type\":\"ConnectorPlacement.EquallySpacedRectSide\",\"uuid\":\"633c2257-0ab1-4a3f-bc19-db971bbd7d23\"},{\"content\":{\"connectorIds\":[\"Out1\"],\"side\":\"RIGHT\"},\"type\":\"ConnectorPlacement.EquallySpacedRectSide\",\"uuid\":\"268aca27-453a-4262-b99b-2b00bb036744\"},{\"content\":{\"connectorIds\":[\"LConn2\"],\"side\":\"TOP\"},\"type\":\"ConnectorPlacement.EquallySpacedRectSide\",\"uuid\":\"94eb7410-69a0-4bb3-bfbc-11fdf2441086\"}]},\"type\":\"ConnectorPlacement.EquallySpacedConnector\",\"uuid\":\"4856a95d-ab29-4fb1-a283-1ba036af507a\"}],\"packageUris\":[\"http://schema.mathworks.com/mf0/Connector/R2020b\"],\"version\":\"1.0\"}"
  DetailedInverter : Subsystem  VariantControl=DetailedOn
      settings: PortSchema="{\"entries\":[{\"content\":{\"sides\":[{\"content\":{\"connectorIds\":[\"In1\",\"In2\",\"LConn1\"]},\"type\":\"ConnectorPlacement.EquallySpacedRectSide\",\"uuid\":\"633c2257-0ab1-4a3f-bc19-db971bbd7d23\"},{\"content\":{\"connectorIds\":[\"Out1\"],\"side\":\"RIGHT\"},\"type\":\"ConnectorPlacement.EquallySpacedRectSide\",\"uuid\":\"268aca27-453a-4262-b99b-2b00bb036744\"},{\"content\":{\"connectorIds\":[\"LConn2\"],\"side\":\"TOP\"},\"type\":\"ConnectorPlacement.EquallySpacedRectSide\",\"uuid\":\"94eb7410-69a0-4bb3-bfbc-11fdf2441086\"}]},\"type\":\"ConnectorPlacement.EquallySpacedConnector\",\"uuid\":\"4856a95d-ab29-4fb1-a283-1ba036af507a\"}],\"packageUris\":[\"http://schema.mathworks.com/mf0/Connector/R2020b\"],\"version\":\"1.0\"}"
  WEGin : PMIOPort  Side=Left
  WEGout : PMIOPort  Port=2  Side=Left
  Tinv : Outport

== system MotorDriveThermalTestbench/Motor Cooling ==
  coolantJacket : Subsystem  VariantControl=JacketOn
  windingOilJet : Subsystem  VariantControl=JetOn
  WindingH : PMIOPort  Side=Left
  JacketH : PMIOPort  Port=2  Side=Left
  Ref : PMIOPort  Port=3  Side=Left

== system MotorDriveThermalTestbench/Subsystem ==
  " " : Inport
  Bus Selector : BusSelector  OutputSignals=Brake pedal,Wind speed,Incline
  PS Gain : fl_lib/Physical Signals/Functions/PS Gain  gain=70 bar
  Simulink-PS Converter : nesl_utility/Simulink-PS Converter  PhysicalDomain=network_engine_domain  SubClassName=ps_input  LeftPortType=input  RightPortType=output  PseudoPeriodic=off  Frequencies=[]  NoiseDistribution=none  NoiseParameters=[]  Unit=1  AffineConversion=off  FilteringAndDerivatives=provide  SimscapeFilterOrder=1  InputFilterTimeConstant=0.001  UdotUserProvided=0
  Simulink-PS Converter1 : nesl_utility/Simulink-PS Converter  PhysicalDomain=network_engine_domain  SubClassName=ps_input  LeftPortType=input  RightPortType=output  PseudoPeriodic=off  Frequencies=[]  NoiseDistribution=none  NoiseParameters=[]  Unit=1  AffineConversion=off  FilteringAndDerivatives=provide  SimscapeFilterOrder=1  InputFilterTimeConstant=0.001  UdotUserProvided=0
  Simulink-PS Converter2 : nesl_utility/Simulink-PS Converter  PhysicalDomain=network_engine_domain  SubClassName=ps_input  LeftPortType=input  RightPortType=output  PseudoPeriodic=off  Frequencies=[]  NoiseDistribution=none  NoiseParameters=[]  Unit=1  AffineConversion=off  FilteringAndDerivatives=provide  SimscapeFilterOrder=1  InputFilterTimeConstant=0.001  UdotUserProvided=0
  wind speed : PMIOPort  Side=Right
  grade : PMIOPort  Port=2  Side=Right
  brk : PMIOPort  Port=3  Side=Right
  wires:
  Bus Selector/1 -> Simulink-PS Converter/1  "<Brake pedal>"
  " "/1 -> Bus Selector/1
  Bus Selector/2 -> Simulink-PS Converter1/1  "<Wind speed>"
  Bus Selector/3 -> Simulink-PS Converter2/1  "<Incline>"
  connections:
  wind speed/RConn1 -- Simulink-PS Converter1/RConn1
  grade/RConn1 -- Simulink-PS Converter2/RConn1
  PS Gain/RConn1 -- brk/RConn1
  PS Gain/LConn1 -- Simulink-PS Converter/RConn1

== system MotorDriveThermalTestbench/TemperatureLimits ==
  Tm : Inport
  Tc : Inport  Port=2
  Tj : Inport  Port=3
  Bus Selector1 : BusSelector  OutputSignals=signal1,signal2
  Mux : Mux  Inputs=2
  Thermal fault Logic Inverter : Subsystem  mask{IGBTlim=448.15, DiodeLim=448.15}
      mask prompts: IGBTlim "IGBT_T_limit(K)"; DiodeLim "Diode_T_Limit(K)"
      mask DialogControl tempCont Prompt: Max T Limits
  Thermal fault Logic Motor : Subsystem  mask{coilTLim=473.15, MagTLim=453.15}
      mask prompts: coilTLim "Coil T Limit"; MagTLim "Mag T Limit"
      mask DialogControl tempCont Prompt: Max T Limits
  fault : Outport
  wires:
  Tj/1 -> Bus Selector1/1
  Tc/1 -> Thermal fault Logic Motor/2(tm)
  Bus Selector1/2 -> Thermal fault Logic Inverter/2(tm)  "<signal2>"
  Thermal fault Logic Inverter/1(F) -> Mux/2
  Thermal fault Logic Motor/1(F) -> Mux/1
  Bus Selector1/1 -> Thermal fault Logic Inverter/1(tc)  "<signal1>"
  Tm/1 -> Thermal fault Logic Motor/1(tc)
  Mux/1 -> fault/1

== system MotorDriveThermalTestbench/Test Env N Controls ==
  Vspd : Inport
  Mspd : Inport  Port=2
  Motor speed N test environment : Subsystem
  Speed Controller : Subsystem
      settings: PortSchema="{\"entries\":[{\"content\":{\"sides\":[{\"content\":{\"connectorIds\":[\"Out1\"]},\"type\":\"ConnectorPlacement.EquallySpacedRectSide\",\"uuid\":\"12b9f2c9-2b28-451b-ad36-7fe4150db485\"},{\"content\":{\"connectorIds\":[\"In1\",\"In2\"],\"side\":\"RIGHT\"},\"type\":\"ConnectorPlacement.EquallySpacedRectSide\",\"uuid\":\"c0fdf9a4-483a-4ddc-b663-6299fcc79327\"},{\"content\":{\"connectorIds\":[],\"side\":\"TOP\"},\"type\":\"ConnectorPlacement.EquallySpacedRectSide\",\"uuid\":\"3f20082e-8487-45e3-9fd7-d6d75741df4d\"}]},\"type\":\"ConnectorPlacement.EquallySpacedConnector\",\"uuid\":\"9361cdd3-74d8-46ee-ae7f-e2dde5d31ed1\"}],\"packageUris\":[\"http://schema.mathworks.com/mf0/Connector/R2020b\"],\"version\":\"1.0\"}"
  TestEnv : Outport
  TorqueCmd : Outport  Port=2
  wires:
  Speed Controller/1(TrqCmd) -> TorqueCmd/1  "TorqueCmd"
  Motor speed N test environment/1(BrakeSig) -> TestEnv/1
  Motor speed N test environment/2(MtrSpdRef) -> Speed Controller/2(SpdRef)
  Vspd/1 -> Motor speed N test environment/1(VehSpd)
  Mspd/1 -> Speed Controller/1(Spd)

== system MotorDriveThermalTestbench/EM/Air_HTC_calculation ==
  Rotor side  HTC : Subsystem
  Rotor_Taylor_Couette  HTC : Subsystem
  w : PMIOPort  Side=Left
  HTC_TC : PMIOPort  Port=2  Side=Right
  HTC : PMIOPort  Port=3  Side=Right
  connections:
  Rotor_Taylor_Couette  HTC/RConn1 -- HTC_TC/RConn1
  HTC/RConn1 -- Rotor side  HTC/RConn1
  Rotor_Taylor_Couette  HTC/LConn1 -- w/RConn1 -- Rotor side  HTC/LConn1

== system MotorDriveThermalTestbench/EM/CurrentMes ==
  Current Sensor : fl_lib/Electrical/Electrical Sensors/Current Sensor
  I : PMIOPort  Side=Left
  + : PMIOPort  Port=2  Side=Left
  - : PMIOPort  Port=3  Side=Right
  connections:
  Current Sensor/LConn1 -- +/RConn1
  Current Sensor/RConn1 -- I/RConn1
  -/RConn1 -- Current Sensor/RConn2

== system MotorDriveThermalTestbench/EM/Loss Estimation ==
  "Copper Loss " : Subsystem
  Iron Loss : Subsystem
  Subsystem : Subsystem
  Hmot : PMIOPort  Side=Left
  I2R : PMIOPort  Port=2  Side=Right
  H_rt : PMIOPort  Port=3  Side=Right
  H_st : PMIOPort  Port=4  Side=Right
  Current : PMIOPort  Port=5  Side=Left
  connections:
  Subsystem/RConn1 -- Iron Loss/LConn1
  I2R/RConn1 -- Iron Loss/LConn2 -- "Copper Loss "/RConn1
  "Copper Loss "/LConn1 -- Current/RConn1
  Hmot/RConn1 -- Subsystem/LConn1
  Iron Loss/RConn2 -- H_st/RConn1
  H_rt/RConn1 -- Iron Loss/RConn1

== system MotorDriveThermalTestbench/EM/Sensing Ref Torque ==
  SL : Inport
  Simulink-PS G1 : nesl_utility/Simulink-PS Converter  PhysicalDomain=network_engine_domain  SubClassName=ps_input  LeftPortType=input  RightPortType=output  PseudoPeriodic=off  Frequencies=[]  NoiseDistribution=none  NoiseParameters=[]  Unit=N*m  AffineConversion=off  FilteringAndDerivatives=zero  SimscapeFilterOrder=1  InputFilterTimeConstant=1e-6  UdotUserProvided=1
  PS : PMIOPort  Side=Right
  wires:
  SL/1 -> Simulink-PS G1/1
  connections:
  Simulink-PS G1/RConn1 -- PS/RConn1

== system MotorDriveThermalTestbench/EM/Speed Measurement ==
  Ideal Rotational Motion Sensor : fl_lib/Mechanical/Mechanical Sensors/Ideal Rotational Motion Sensor  reference=foundation.enum.MeasurementReference.difference  acceleration_port=false  velocity_port=true  position_port=false  wrap_angle=false  offset=0 rad
      settings: InternalSimscapePortConfiguration="{\"Bottom\":[],\"Left\":[{\"id\":\"R\",\"label\":\"R\",\"type\":\"foundation.mechanical.rotational.rotational\"}],\"Right\":[{\"id\":\"C\",\"label\":\"C\",\"type\":\"foundation.mechanical.rotational.rotational\"},{\"id\":\"W\",\"label\":\"W\",\"type\":\"output\"}],\"Top\":[]}"
  MRRef1 : fl_lib/Mechanical/Rotational Elements/Mechanical Rotational Reference
  spd : PMIOPort  Side=Right
  mot : PMIOPort  Port=2  Side=Left
  connections:
  spd/RConn1 -- Ideal Rotational Motion Sensor/RConn2
  mot/RConn1 -- Ideal Rotational Motion Sensor/LConn1
  MRRef1/LConn1 -- Ideal Rotational Motion Sensor/RConn1

== system MotorDriveThermalTestbench/EM/Subsystem1 ==
  Sensing wMotor : Subsystem
      mask Display: disp('w');
  PS : PMIOPort  Side=Left
  w : Outport  VectorParamsAs1DForOutWhenUnconnected=off
  wires:
  Sensing wMotor/1(SL) -> w/1
  connections:
  PS/RConn1 -- Sensing wMotor/LConn1

== system MotorDriveThermalTestbench/EM/Temperature ==
  Bus : Subsystem
  Rotor Thermal Block : Subsystem
  Stator Thermal Block : Subsystem
  I2R : PMIOPort  Side=Left
  H_rt : PMIOPort  Port=2  Side=Left
  H_st : PMIOPort  Port=3  Side=Left
  HTC_TC : PMIOPort  Port=4  Side=Left
  HTC : PMIOPort  Port=5  Side=Left
  Hjacket : PMIOPort  Port=6  Side=Right
  Hwinding : PMIOPort  Port=7  Side=Right
  Tmot : Outport
  wires:
  Bus/1("   ") -> Tmot/1
  connections:
  Hwinding/RConn1 -- Stator Thermal Block/LConn3
  Stator Thermal Block/LConn1 -- Bus/LConn2
  Rotor Thermal Block/LConn1 -- Bus/LConn1
  HTC/RConn1 -- Rotor Thermal Block/RConn3
  HTC_TC/RConn1 -- Rotor Thermal Block/RConn2
  I2R/RConn1 -- Stator Thermal Block/RConn2
  H_st/RConn1 -- Stator Thermal Block/RConn1
  H_rt/RConn1 -- Rotor Thermal Block/RConn1
  Hjacket/RConn1 -- Stator Thermal Block/LConn2

== system MotorDriveThermalTestbench/Inverter/AbstractInverter  ==
  mspd : Inport
  mtrq : Inport  Port=2
  Inverter Power Module Thermal : Subsystem
  WEGin : PMIOPort  Side=Left
  WEGout : PMIOPort  Port=2  Side=Left
  Tinv : Outport
  wires:
  mtrq/1 -> Inverter Power Module Thermal/2(motorTrq)
  Inverter Power Module Thermal/1(InverterT) -> Tinv/1
  mspd/1 -> Inverter Power Module Thermal/1(motorSpd)
  connections:
  WEGin/RConn1 -- Inverter Power Module Thermal/LConn1
  WEGout/RConn1 -- Inverter Power Module Thermal/RConn1

== system MotorDriveThermalTestbench/Inverter/DetailedInverter ==
  mspd : Inport
  mtrq : Inport  Port=2
  BaseplateAndHeatsink : Subsystem
      settings: PortSchema="{\"entries\":[{\"content\":{\"sides\":[{\"content\":{\"connectorIds\":[\"LConn1\"]},\"type\":\"ConnectorPlacement.EquallySpacedRectSide\",\"uuid\":\"e581cfdc-799f-4cc5-addf-0469cfe4cea9\"},{\"content\":{\"connectorIds\":[\"RConn1\",\"Out1\"],\"side\":\"RIGHT\"},\"type\":\"ConnectorPlacement.EquallySpacedRectSide\",\"uuid\":\"aa2a4c2d-5a60-4c16-854d-0ab5d1d8d47e\"},{\"content\":{\"connectorIds\":[\"LConn2\"],\"side\":\"TOP\"},\"type\":\"ConnectorPlacement.EquallySpacedRectSide\",\"uuid\":\"f95ebc04-b810-4731-a06d-2fefe276a00e\"}]},\"type\":\"ConnectorPlacement.EquallySpacedConnector\",\"uuid\":\"dfaa3921-5b0c-4412-88f7-1b42ae388064\"}],\"packageUris\":[\"http://schema.mathworks.com/mf0/Connector/R2020b\"],\"version\":\"1.0\"}"
  Bus Creator : BusCreator  Inputs=2
  PowerLoss : Subsystem
      settings: PortSchema="{\"entries\":[{\"content\":{\"sides\":[{\"content\":{\"connectorIds\":[\"In1\",\"In2\"]},\"type\":\"ConnectorPlacement.EquallySpacedRectSide\",\"uuid\":\"127a6954-bfd2-4a2c-bf6e-1fabee693a74\"},{\"content\":{\"connectorIds\":[\"Out1\",\"Out2\"],\"side\":\"RIGHT\"},\"type\":\"ConnectorPlacement.EquallySpacedRectSide\",\"uuid\":\"d7114e53-5a47-441c-8b7e-c8f7f7446772\"},{\"content\":{\"connectorIds\":[\"In3\",\"In4\"],\"side\":\"TOP\"},\"type\":\"ConnectorPlacement.EquallySpacedRectSide\",\"uuid\":\"b7197b4d-20b7-4d66-a096-8a3dac2059b0\"}]},\"type\":\"ConnectorPlacement.EquallySpacedConnector\",\"uuid\":\"cbecf243-309a-43cf-9150-c3824f42fd07\"}],\"packageUris\":[\"http://schema.mathworks.com/mf0/Connector/R2020b\"],\"version\":\"1.0\"}"
  Scope : Scope
  Scope1 : Scope
  Switches : Subsystem  VariantControl=Reduced - Use only for thermal steady-state estimation
      settings: PortSchema="{\"entries\":[{\"content\":{\"sides\":[{\"content\":{\"connectorIds\":[]},\"type\":\"ConnectorPlacement.EquallySpacedRectSide\",\"uuid\":\"13dd74a1-5c62-48c5-9ddb-fd86d3425da3\"},{\"content\":{\"connectorIds\":[\"RConn1\"],\"side\":\"RIGHT\"},\"type\":\"ConnectorPlacement.EquallySpacedRectSide\",\"uuid\":\"5f5f3d4d-e36b-4884-95be-8fef19471975\"},{\"content\":{\"connectorIds\":[\"Out1\",\"Out2\"],\"side\":\"TOP\"},\"type\":\"ConnectorPlacement.EquallySpacedRectSide\",\"uuid\":\"81739398-d25c-47c6-bb27-3c5556be241b\"},{\"content\":{\"connectorIds\":[\"In1\",\"In2\"],\"side\":\"BOTTOM\"},\"type\":\"ConnectorPlacement.EquallySpacedRectSide\",\"uuid\":\"53853fa3-d12c-4a2a-8100-cc62f56e0a4a\"}]},\"type\":\"ConnectorPlacement.EquallySpacedConnector\",\"uuid\":\"007acc50-585e-47a3-b589-6267a8a6c1c2\"}],\"packageUris\":[\"http://schema.mathworks.com/mf0/Connector/R2020b\"],\"version\":\"1.0\"}"
      mask Display: image('$imagefile'); % Use "Edit Image" on toolstrip to change.
  WEGin : PMIOPort  Side=Left
  WEGout : PMIOPort  Port=2  Side=Left
  Tinv : Outport
  wires:
  Bus Creator/1 -> Scope1/1, Tinv/1
  mspd/1 -> PowerLoss/1(mspd)
  mtrq/1 -> PowerLoss/2(tq)
  Switches/1(Ti) -> PowerLoss/4(Tigbt), Bus Creator/1
  PowerLoss/1(Higbt) -> Switches/1(HI)
  PowerLoss/2(Hdiode) -> Switches/2(HD)
  Switches/2(Td) -> Bus Creator/2, PowerLoss/3(Tdiode)
  BaseplateAndHeatsink/1(Tc) -> Scope/1
  connections:
  Switches/RConn1 -- BaseplateAndHeatsink/LConn2
  WEGout/RConn1 -- BaseplateAndHeatsink/RConn1
  WEGin/RConn1 -- BaseplateAndHeatsink/LConn1
